simulink model "Simscape_DC_Motor_SPE_START"  (R2014a)
settings: Solver=ode15s  StartTime=0.0  StopTime=4  RelTol=1e-3
PreLoadFcn:
  | load Simscape_DC_Motor_SPE_Data;
  | load Simscape_DC_Motor_SPE_Param_Start;
values from neighbouring files (symbols this model uses):
  DC_Motor_B = 1.07154447217    [Simscape_DC_Motor_SPE_Param_Final.mat]
  DC_Motor_K = 0.453596339369    [Simscape_DC_Motor_SPE_Param_Final.mat]
  DC_Motor_R = 4.03046032748    [Simscape_DC_Motor_SPE_Param_Final.mat]
libraries: fl_lib x22, nesl_utility x6
Description:
  | Copyright 2014 The MathWorks, Inc.
settings Model: Creator=smiller  LastModifiedBy=smiller
settings DataIOCC: ExternalInput=[SS_DC_Motor_SPE_Input_time SS_DC_Motor_SPE_Input_Signal]  LoadExternalInput=on
settings OptimizationCC: ExpressionDepthLimit=2147483647  InitFltsAndDblsToZero=on
settings DebuggingCC: SaveWithParameterizedLinksMsg=none  UnderspecifiedInitializationDetection=Classic  SolverPrmCheckMsg=none  FcnCallInpInsideContextMsg=UseLocalSettings  StateNameClashWarn=warning
settings GRTTargetCC: TargetFcnLib=ansi_tfl_tmw.mat  CombineOutputUpdateFcns=off  GRTInterface=on

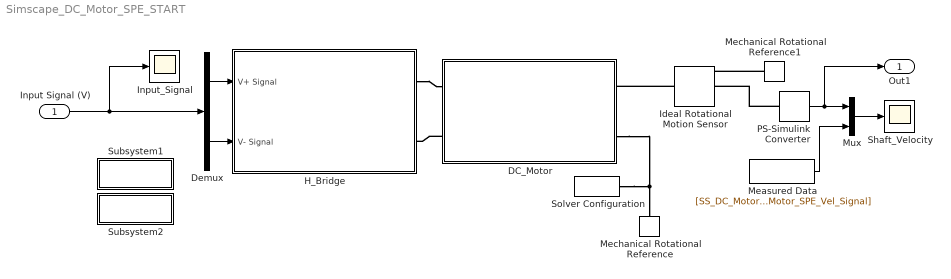
== system Simscape_DC_Motor_SPE_START ==
  Input Signal (V) : Inport  PortDimensions=2
  DC_Motor : Subsystem
      mask Display:
      | image(imread('Simscape_DC_Motor.jpg'));
      | port_label('lconn',1,'V+');
      | port_label('lconn',2,'V-');
      | port_label('rconn',1,'Shaft');
      | port_label('rconn',2,'Housing');
  Demux : Demux  Outputs=2
  H_Bridge : Subsystem
      mask Display:
      | image(imread('H_Bridge.jpg'));
      | port_label('Input',1,'V+ Signal');
      | port_label('Input',2,'V- Signal');
      | port_label('rconn',1,'V+');
      | port_label('rconn',2,'V-');
  Ideal Rotational Motion Sensor : fl_lib/Mechanical/Mechanical Sensors/Ideal Rotational Motion Sensor  offset=0 rad
  Input_Signal : Scope
      settings: YMin=-0.5  YMax=1.5  SaveName=PWin_SPE_Input_Signal
  Measured Data : FromWorkspace  VariableName=[SS_DC_Motor_SPE_Vel_time SS_DC_Motor_SPE_Vel_Signal]  SampleTime=0
  Mechanical Rotational Reference : fl_lib/Mechanical/Rotational Elements/Mechanical Rotational Reference
  Mechanical Rotational Reference1 : fl_lib/Mechanical/Rotational Elements/Mechanical Rotational Reference
  Mux : Mux  Inputs=2
  PS-Simulink Converter : nesl_utility/PS-Simulink Converter  PhysicalDomain=network_engine_domain  SubClassName=ps_output  LeftPortType=input  RightPortType=output  PseudoPeriodic=off  Frequencies=[]  Unit=1  AffineConversion=off
  Shaft_Velocity : Scope
      settings: YMin=-1.5  YMax=1.5  SaveName=SS_DC_Motor_SPE_DATA
  Solver Configuration : nesl_utility/Solver Configuration  PhysicalDomain=network_engine_domain  SubClassName=solver  LeftPortType=input  RightPortType=generic  Accelerate=off  Tones=[]  Harmonics=[]  SimulateNoise=off  Profile=off  UseLocalSampling=off  EnableSwitchedLinearOptims=on  FrequencyDomain=off  UseCCode=off  RelTol=0.001  AbsTol=1e-06  MinStep=1e-09  ToWorkspace=off  DoDC=off  ResidualTolerance=1e-9  UseLocalSolver=off  LocalSolverChoice=NE_BACKWARD_EULER_ADVANCER  LocalSolverSampleTime=.001  DoFixedCost=off  MaxNonlinIter=12  MaxModeIter=1  LinearAlgebra=Sparse  DelaysMemoryBudget=1024  AutomaticFiltering=on  FilteringTimeConstant=0.001
  Subsystem1 : Subsystem
      settings: OpenFcn=load Simscape_DC_Motor_SPE_Param_Start;
      mask Display: disp('Orig. Values')
  Subsystem2 : Subsystem
      settings: OpenFcn=load Simscape_DC_Motor_SPE_Param_Final;
      mask Display: disp('Final Values')
  Out1 : Outport
  wires:
  Input Signal (V)/1 -> Demux/1, Input_Signal/1
  Demux/1 -> H_Bridge/1(V+ Signal)
  Demux/2 -> H_Bridge/2(V- Signal)
  Mux/1 -> Shaft_Velocity/1
  Measured Data/1 -> Mux/2
  PS-Simulink Converter/1 -> Out1/1, Mux/1
  connections:
  DC_Motor/RConn2 -- Mechanical Rotational Reference/LConn1 -- Solver Configuration/RConn1
  Ideal Rotational Motion Sensor/LConn1 -- DC_Motor/RConn1
  Mechanical Rotational Reference1/LConn1 -- Ideal Rotational Motion Sensor/RConn1
  PS-Simulink Converter/LConn1 -- Ideal Rotational Motion Sensor/RConn2
  H_Bridge/RConn1 -- DC_Motor/LConn1
  DC_Motor/LConn2 -- H_Bridge/RConn2

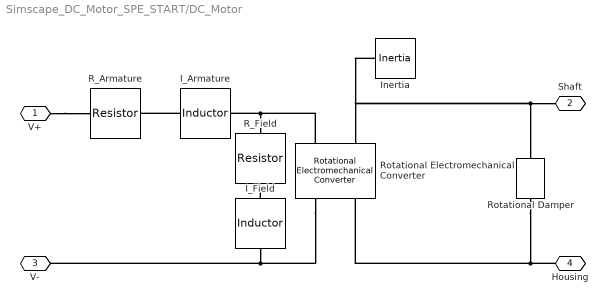
== system Simscape_DC_Motor_SPE_START/DC_Motor ==
  I_Armature : fl_lib/Electrical/Electrical Elements/Inductor  l=DC_Motor_L H  r=0 Ohm  g=1e-09 1/Ohm  i_specify=off  i_priority=High  i=0 A  v_specify=off  v_priority=High  v=0 V  i_L_specify=on  i_L_priority=High  i_L=0 A
  I_Field : fl_lib/Electrical/Electrical Elements/Inductor  l=1e-6 H  r=0 Ohm  g=1e-09 1/Ohm  i_specify=off  i_priority=High  i=0 A  v_specify=off  v_priority=High  v=0 V  i_L_specify=on  i_L_priority=High  i_L=0 A
  Inertia : fl_lib/Mechanical/Rotational Elements/Inertia  inertia=DC_Motor_J kg*m^2  w_specify=on  w_priority=High  w=0 rad/s  t_specify=off  t_priority=High  t=0 N*m
  R_Armature : fl_lib/Electrical/Electrical Elements/Resistor  R=DC_Motor_R Ohm  i_specify=off  i_priority=High  i=0 A  v_specify=off  v_priority=High  v=0 V
  R_Field : fl_lib/Electrical/Electrical Elements/Resistor  R=1e6 Ohm  i_specify=off  i_priority=High  i=0 A  v_specify=off  v_priority=High  v=0 V
  Rotational Damper : fl_lib/Mechanical/Rotational Elements/Rotational Damper  D=DC_Motor_B N*m/(rad/s)  w_specify=off  w_priority=High  w=0 rad/s  t_specify=off  t_priority=High  t=0 N*m
  Rotational Electromechanical Converter : fl_lib/Electrical/Electrical Elements/Rotational Electromechanical Converter  K=DC_Motor_K V/(rad/s)  i_specify=off  i_priority=High  i=0 A  v_specify=off  v_priority=High  v=0 V  t_specify=off  t_priority=High  t=0 N*m  w_specify=off  w_priority=High  w=0 rad/s
  V+ : PMIOPort  Port=1  Side=Left
  Shaft : PMIOPort  Port=2  Side=Right
  V- : PMIOPort  Port=3  Side=Left
  Housing : PMIOPort  Port=4  Side=Right
  connections:
  I_Armature/LConn1 -- R_Armature/RConn1
  Rotational Electromechanical Converter/LConn1 -- I_Armature/RConn1 -- R_Field/LConn1
  Rotational Electromechanical Converter/RConn1 -- V-/RConn1 -- I_Field/RConn1
  Rotational Electromechanical Converter/LConn2 -- Inertia/LConn1 -- Shaft/RConn1 -- Rotational Damper/LConn1
  V+/RConn1 -- R_Armature/LConn1
  Housing/RConn1 -- Rotational Electromechanical Converter/RConn2 -- Rotational Damper/RConn1
  I_Field/LConn1 -- R_Field/RConn1

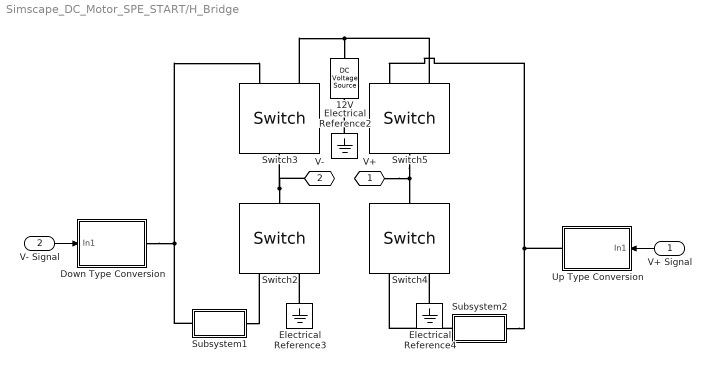
== system Simscape_DC_Motor_SPE_START/H_Bridge ==
  V+ Signal : Inport
  V- Signal : Inport  Port=2
  12V : fl_lib/Electrical/Electrical Sources/DC Voltage Source  v0=12 V
  Down Type Conversion : Subsystem
  Electrical Reference2 : fl_lib/Electrical/Electrical Elements/Electrical Reference
  Electrical Reference3 : fl_lib/Electrical/Electrical Elements/Electrical Reference
  Electrical Reference4 : fl_lib/Electrical/Electrical Elements/Electrical Reference
  Subsystem1 : Subsystem
      mask Display: disp('NOT');
  Subsystem2 : Subsystem
      mask Display: disp('NOT');
  Switch{2..5} (4 alike) : fl_lib/Electrical/Electrical Elements/Switch  R_closed=0.01 Ohm  G_open=1e-8 1/Ohm  Threshold=0  i_specify=off  i_priority=High  i=0 A  v_specify=off  v_priority=High  v=0 V
  Up Type Conversion : Subsystem
  V+ : PMIOPort  Port=1  Side=Right
  V- : PMIOPort  Port=2  Side=Right
  wires:
  V+ Signal/1 -> Up Type Conversion/1(In1)
  V- Signal/1 -> Down Type Conversion/1(In1)
  connections:
  Up Type Conversion/RConn1 -- Switch5/RConn1 -- Subsystem2/LConn1
  Subsystem2/RConn1 -- Switch4/RConn1
  Electrical Reference4/LConn1 -- Switch4/RConn2
  Subsystem1/RConn1 -- Switch2/RConn1
  Electrical Reference3/LConn1 -- Switch2/RConn2
  Electrical Reference2/LConn1 -- 12V/RConn1
  Switch2/LConn1 -- Switch3/LConn1 -- V-/RConn1
  Down Type Conversion/RConn1 -- Switch3/RConn1 -- Subsystem1/LConn1
  Switch5/RConn2 -- 12V/LConn1 -- Switch3/RConn2
  Switch5/LConn1 -- Switch4/LConn1 -- V+/RConn1

== system Simscape_DC_Motor_SPE_START/Subsystem1 ==

== system Simscape_DC_Motor_SPE_START/Subsystem2 ==

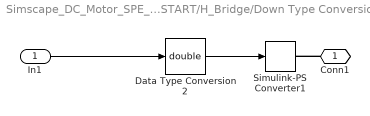
== system Simscape_DC_Motor_SPE_START/H_Bridge/Down Type Conversion ==
  In1 : Inport
  Data Type Conversion2 : DataTypeConversion  OutDataTypeStr=double
  Simulink-PS Converter1 : nesl_utility/Simulink-PS Converter  PhysicalDomain=network_engine_domain  SubClassName=ps_input  LeftPortType=input  RightPortType=output  PseudoPeriodic=off  Frequencies=[]  NoiseDistribution=none  NoiseParameters=[]  Unit=1  AffineConversion=off  InputFiltering=off  SimscapeFilterOrder=1  InputFilterTimeConstant=.001  UdotUserProvided=0
  Conn1 : PMIOPort  Port=1  Side=Right
  wires:
  Data Type Conversion2/1 -> Simulink-PS Converter1/1
  In1/1 -> Data Type Conversion2/1
  connections:
  Conn1/RConn1 -- Simulink-PS Converter1/RConn1

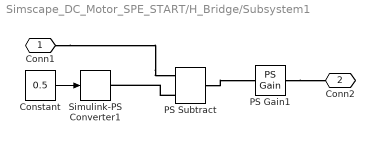
== system Simscape_DC_Motor_SPE_START/H_Bridge/Subsystem1 ==
  Constant : Constant  Value=0.5
  PS Gain1 : fl_lib/Physical Signals/Functions/PS Gain  gain=-1
  PS Subtract : fl_lib/Physical Signals/Functions/PS Subtract
  Simulink-PS Converter1 : nesl_utility/Simulink-PS Converter  PhysicalDomain=network_engine_domain  SubClassName=ps_input  LeftPortType=input  RightPortType=output  PseudoPeriodic=off  Frequencies=[]  NoiseDistribution=none  NoiseParameters=[]  Unit=1  AffineConversion=off  InputFiltering=off  SimscapeFilterOrder=1  InputFilterTimeConstant=.001  UdotUserProvided=0
  Conn1 : PMIOPort  Port=1  Side=Left
  Conn2 : PMIOPort  Port=2  Side=Right
  wires:
  Constant/1 -> Simulink-PS Converter1/1
  connections:
  PS Subtract/LConn2 -- Simulink-PS Converter1/RConn1
  Conn1/RConn1 -- PS Subtract/LConn1
  PS Subtract/RConn1 -- PS Gain1/LConn1
  PS Gain1/RConn1 -- Conn2/RConn1

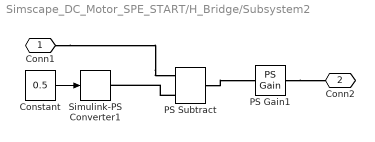
== system Simscape_DC_Motor_SPE_START/H_Bridge/Subsystem2 ==
  Constant : Constant  Value=0.5
  PS Gain1 : fl_lib/Physical Signals/Functions/PS Gain  gain=-1
  PS Subtract : fl_lib/Physical Signals/Functions/PS Subtract
  Simulink-PS Converter1 : nesl_utility/Simulink-PS Converter  PhysicalDomain=network_engine_domain  SubClassName=ps_input  LeftPortType=input  RightPortType=output  PseudoPeriodic=off  Frequencies=[]  NoiseDistribution=none  NoiseParameters=[]  Unit=1  AffineConversion=off  InputFiltering=off  SimscapeFilterOrder=1  InputFilterTimeConstant=.001  UdotUserProvided=0
  Conn1 : PMIOPort  Port=1  Side=Left
  Conn2 : PMIOPort  Port=2  Side=Right
  wires:
  Constant/1 -> Simulink-PS Converter1/1
  connections:
  PS Gain1/RConn1 -- Conn2/RConn1
  PS Subtract/RConn1 -- PS Gain1/LConn1
  Conn1/RConn1 -- PS Subtract/LConn1
  PS Subtract/LConn2 -- Simulink-PS Converter1/RConn1

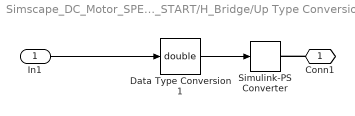
== system Simscape_DC_Motor_SPE_START/H_Bridge/Up Type Conversion ==
  In1 : Inport
  Data Type Conversion1 : DataTypeConversion  OutDataTypeStr=double
  Simulink-PS Converter : nesl_utility/Simulink-PS Converter  PhysicalDomain=network_engine_domain  SubClassName=ps_input  LeftPortType=input  RightPortType=output  PseudoPeriodic=off  Frequencies=[]  NoiseDistribution=none  NoiseParameters=[]  Unit=1  AffineConversion=off  InputFiltering=off  SimscapeFilterOrder=1  InputFilterTimeConstant=.001  UdotUserProvided=0
  Conn1 : PMIOPort  Port=1  Side=Right
  wires:
  Data Type Conversion1/1 -> Simulink-PS Converter/1
  In1/1 -> Data Type Conversion1/1
  connections:
  Conn1/RConn1 -- Simulink-PS Converter/RConn1
